simulink model "Feedback_Configuration_1"  (R2021b)
settings: Solver=VariableStepAuto  StartTime=0.0  StopTime=24.00  RelTol=1e-3
values from neighbouring files (symbols this model uses):
  R = 1.15    [pratica6.m]
libraries: cstblocks x8
settings Model: Creator=carlo  LastModifiedBy=carlo

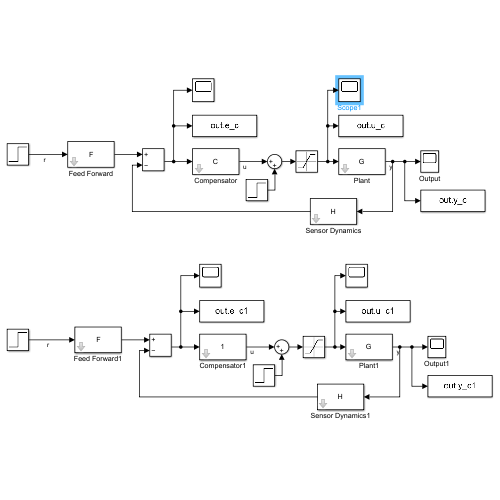
[thumbnail: Simulink's stored preview of the top-level diagram]
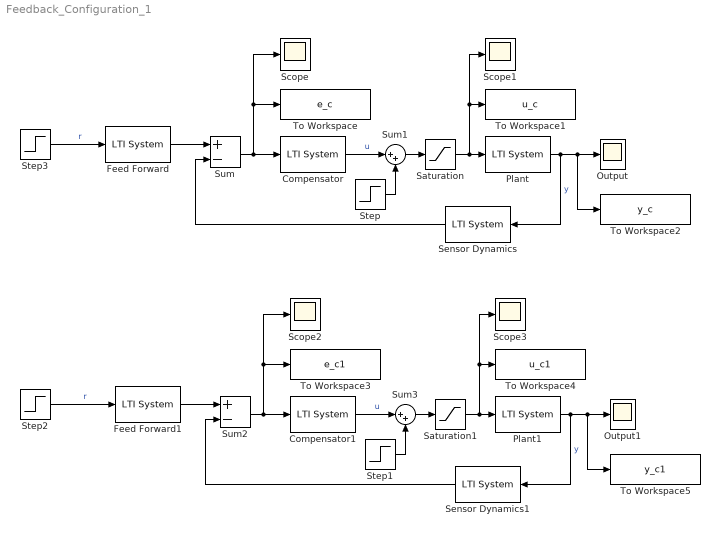
== system Feedback_Configuration_1 ==
  Compensator : cstblocks/LTI System  sys=C  IC=[]
  Compensator1 : cstblocks/LTI System  sys=1  IC=[]
  Feed Forward : cstblocks/LTI System  sys=F  IC=[]
  Feed Forward1 : cstblocks/LTI System  sys=F  IC=[]
  Output : Scope
  Output1 : Scope
  Plant : cstblocks/LTI System  sys=G  IC=[]
  Plant1 : cstblocks/LTI System  sys=G  IC=[]
  Saturation : Saturate  UpperLimit=10  LowerLimit=-10
  Saturation1 : Saturate  UpperLimit=10  LowerLimit=-10
  Scope{,1..3} (4 alike) : Scope
  Sensor Dynamics : cstblocks/LTI System  sys=H  IC=[]
  Sensor Dynamics1 : cstblocks/LTI System  sys=H  IC=[]
  Step : Step  Time=12  After=0.26  SampleTime=0
  Step1 : Step  Time=12  After=0.26  SampleTime=0
  Step2 : Step  Time=0  After=R  SampleTime=0
  Step3 : Step  Time=0  After=R  SampleTime=0
  Sum : Sum  Inputs=+-
  Sum1 : Sum  Inputs=|++
  Sum2 : Sum  Inputs=+-
  Sum3 : Sum  Inputs=|++
  To Workspace : ToWorkspace  VariableName=e_c  SaveFormat=Timeseries  SampleTime=-1
  To Workspace1 : ToWorkspace  VariableName=u_c  SaveFormat=Timeseries  SampleTime=-1
  To Workspace2 : ToWorkspace  VariableName=y_c  SaveFormat=Timeseries  SampleTime=-1
  To Workspace3 : ToWorkspace  VariableName=e_c1  SaveFormat=Timeseries  SampleTime=-1
  To Workspace4 : ToWorkspace  VariableName=u_c1  SaveFormat=Timeseries  SampleTime=-1
  To Workspace5 : ToWorkspace  VariableName=y_c1  SaveFormat=Timeseries  SampleTime=-1
  wires:
  Step3/1 -> Feed Forward/1  "r"
  Feed Forward/1 -> Sum/1
  Sensor Dynamics/1 -> Sum/2
  Sum/1 -> Compensator/1, To Workspace/1, Scope/1
  Compensator/1 -> Sum1/1  "u"
  Plant/1 -> To Workspace2/1, Output/1, Sensor Dynamics/1  "y"
  Sum1/1 -> Saturation/1
  Step/1 -> Sum1/2
  Saturation/1 -> To Workspace1/1, Scope1/1, Plant/1
  Plant1/1 -> To Workspace5/1, Output1/1, Sensor Dynamics1/1  "y"
  Sum2/1 -> Compensator1/1, To Workspace3/1, Scope2/1
  Compensator1/1 -> Sum3/1  "u"
  Step2/1 -> Feed Forward1/1  "r"
  Feed Forward1/1 -> Sum2/1
  Step1/1 -> Sum3/2
  Sensor Dynamics1/1 -> Sum2/2
  Sum3/1 -> Saturation1/1
  Saturation1/1 -> To Workspace4/1, Scope3/1, Plant1/1
